simulink model "CAVLAB"  (R2019a)
settings: Solver=FixedStepAuto  StartTime=0.0  StopTime=3888000  FixedStep=3600  RelTol=1e-3
settings Model: Creator=Afaq  LastModifiedBy=Afaq

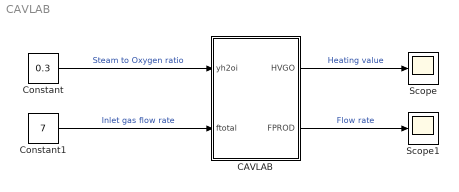
== system CAVLAB ==
  "CAVLAB " : Subsystem
  Constant : Constant  Value=0.3
  Constant1 : Constant  Value=7
  Scope : Scope
  Scope1 : Scope
  wires:
  "CAVLAB "/1(HVGO) -> Scope/1  "Heating value"
  "CAVLAB "/2(FPROD) -> Scope1/1  "Flow rate"
  Constant/1 -> "CAVLAB "/1("yh2oi ")  "Steam to Oxygen ratio"
  Constant1/1 -> "CAVLAB "/2(ftotal)  "Inlet gas flow rate"

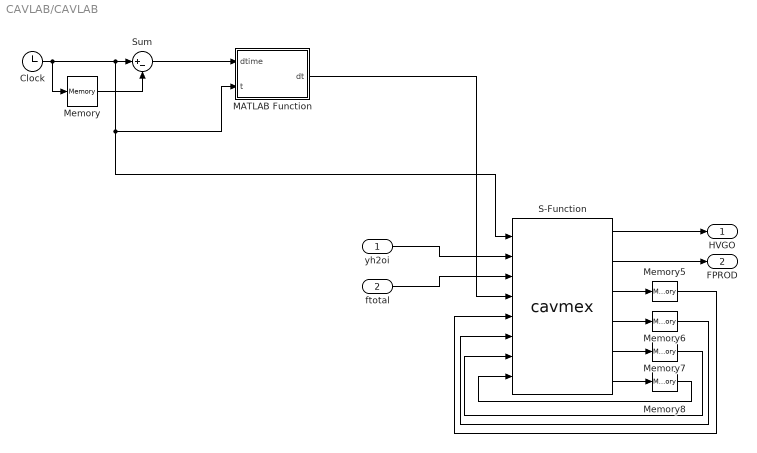
== system CAVLAB/CAVLAB  ==
  "yh2oi " : Inport
  ftotal : Inport  Port=2
  Clock : Clock
  MATLAB Function : MATLAB Function  TreatAsAtomicUnit=on
  Memory{,5..8} (5 alike) : Memory
  S-Function : S-Function  FunctionName=cavmex  SFunctionDeploymentMode=off  EnableBusSupport=off
  Sum : Sum  Inputs=|+-
  HVGO : Outport
  FPROD : Outport  Port=2
  wires:
  Clock/1 -> Memory/1, S-Function/1, MATLAB Function/2(t), Sum/1
  Memory/1 -> Sum/2
  S-Function/3 -> Memory5/1
  S-Function/4 -> Memory6/1
  S-Function/5 -> Memory7/1
  S-Function/6 -> Memory8/1
  Memory8/1 -> S-Function/8
  Memory7/1 -> S-Function/7
  Memory6/1 -> S-Function/6
  Memory5/1 -> S-Function/5
  ftotal/1 -> S-Function/3
  "yh2oi "/1 -> S-Function/2
  Sum/1 -> MATLAB Function/1(dtime)
  S-Function/1 -> HVGO/1
  S-Function/2 -> FPROD/1
  MATLAB Function/1(dt) -> S-Function/4

== matlab function CAVLAB/CAVLAB /MATLAB Function ==
  data: dtime input; t input; dt output
function dt = fcn(dtime,t)
if t<=3600
    dt=dtime;
else
    dt=dtime;
end
end
